simulink model "CurrentKalmanTest"  (R2015a)
settings: Solver=ode45  StartTime=0.0  StopTime=50  RelTol=1e-3
undefined symbols (not defined in the file or in its folder): Continuous, Time
libraries: ctrlSharedLib x1
settings Model: Creator=jinkale  LastModifiedBy=jinkale

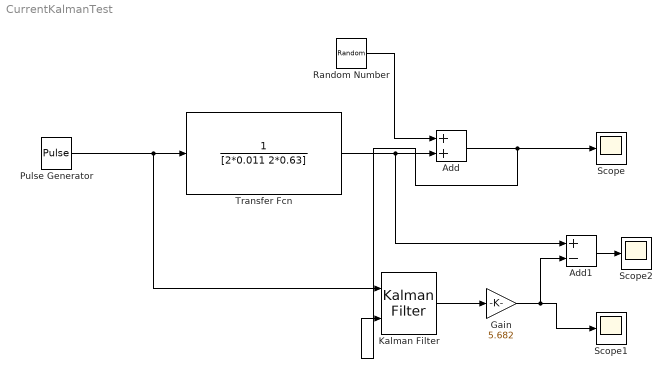
== system CurrentKalmanTest ==
  Add : Sum
  Add1 : Sum  Inputs=+-
  Gain : Gain  Gain=5.682
  Kalman Filter : ctrlSharedLib/Kalman Filter  TimeDomain=Continuous-Time  UseCurrentEstimator=on  ModelSource=Individual A, B, C, D matrices  ModelSourceVariable=ss(0.95,1,1,0,1)  A=-57.27  B=8  C=5.682  D=0  NumberOfStates=1  NumberOfInputs=1  NumberOfOutputs=1  InitialEstimateSource=Dialog  X0=0  P0=10  UseK=off  UseGH=off  NumberOfProcessNoiseInputs=1  G=1  TimeInvariantG=on  H=0  TimeInvariantH=on  Q=0.000001  TimeInvariantQ=on  R=0.036  TimeInvariantR=on  N=0  TimeInvariantN=on  AddInputPort=on  AddEnablePort=off  OutputEstimatedY=off  OutputP=off  Ts=-1
  Pulse Generator : DiscretePulseGenerator  PulseType=Time based  Amplitude=3  Period=10  PulseWidth=50
  Random Number : RandomNumber  Variance=0.0360  SampleTime=1/200
  Scope : Scope
  Scope1 : Scope
  Scope2 : Scope
      settings: SaveName=ScopeData2
  Transfer Fcn : TransferFcn  Denominator=[2*0.011 2*0.63]
  wires:
  Pulse Generator/1 -> Kalman Filter/1, Transfer Fcn/1
  Random Number/1 -> Add/1
  Transfer Fcn/1 -> Add1/1, Add/2
  Add/1 -> Kalman Filter/2, Scope/1
  Add1/1 -> Scope2/1
  Kalman Filter/1 -> Gain/1
  Gain/1 -> Add1/2, Scope1/1
